simulink model "stepResponseModel"  (R2015a)
settings: Solver=ode45  StartTime=0.0  StopTime=simulationTime  RelTol=1e-3
values from neighbouring files (symbols this model uses):
  u1_fin = U(1,2)    [SVDecomp.m]    (also in stepResponse.m = 0)
  u2_fin = U(2,2)    [SVDecomp.m]    (also in stepResponse.m = 1)
settings Model: Creator=bram  LastModifiedBy=bram

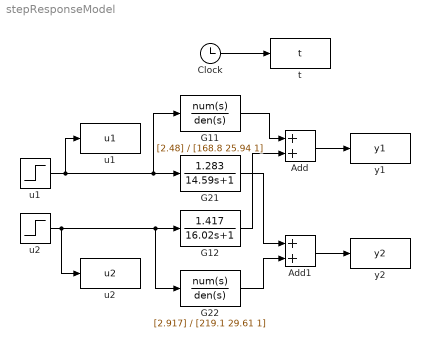
== system stepResponseModel ==
  Add : Sum
  Add1 : Sum
  Clock : Clock
  G11 : TransferFcn  Numerator=[2.48]  Denominator=[168.8 25.94 1]
  G12 : TransferFcn  Numerator=[1.417]  Denominator=[16.02 1]
  G21 : TransferFcn  Numerator=[1.283]  Denominator=[14.59 1]
  G22 : TransferFcn  Numerator=[2.917]  Denominator=[219.1 29.61 1]
  t : ToWorkspace  VariableName=t  SampleTime=-1
  u1 : Step  Time=100  After=u1_fin  SampleTime=0
  "u1 " : ToWorkspace  VariableName=u1  SampleTime=-1
  u2 : Step  Time=100  After=u2_fin  SampleTime=0
  "u2 " : ToWorkspace  VariableName=u2  SampleTime=-1
  y1 : ToWorkspace  VariableName=y1  SampleTime=-1
  y2 : ToWorkspace  VariableName=y2  SampleTime=-1
  wires:
  u1/1 -> "u1 "/1, G21/1, G11/1
  u2/1 -> "u2 "/1, G22/1, G12/1
  G21/1 -> Add1/1
  G22/1 -> Add1/2
  G12/1 -> Add/2
  G11/1 -> Add/1
  Add/1 -> y1/1
  Add1/1 -> y2/1
  Clock/1 -> t/1
